simulink model "linearExtendedStateObserver"  (R2021a)
settings: Solver=VariableStepAuto  StartTime=0.0  StopTime=10.0  RelTol=1e-3
settings Model: Creator=krzys  LastModifiedBy=krzys

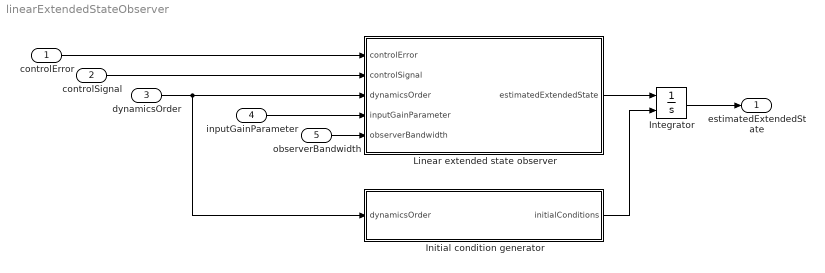
== system linearExtendedStateObserver ==
  controlError : Inport
  controlSignal : Inport  Port=2
  dynamicsOrder : Inport  Port=3
  inputGainParameter : Inport  Port=4
  observerBandwidth : Inport  Port=5
  Initial condition generator : MATLAB Function  TreatAsAtomicUnit=on
  Integrator : Integrator  InitialConditionSource=external
  Linear extended state observer : MATLAB Function  TreatAsAtomicUnit=on
  estimatedExtendedState : Outport
  wires:
  controlError/1 -> Linear extended state observer/1(controlError)
  controlSignal/1 -> Linear extended state observer/2(controlSignal)
  Linear extended state observer/1(estimatedExtendedState) -> Integrator/1
  Integrator/1 -> estimatedExtendedState/1
  dynamicsOrder/1 -> Initial condition generator/1(dynamicsOrder), Linear extended state observer/3(dynamicsOrder)
  inputGainParameter/1 -> Linear extended state observer/4(inputGainParameter)
  observerBandwidth/1 -> Linear extended state observer/5(observerBandwidth)
  Initial condition generator/1(initialConditions) -> Integrator/2

== matlab function linearExtendedStateObserver/Initial condition generator ==
  data: dynamicsOrder input; initialConditions output
function initialConditions = fcn(dynamicsOrder)
    initialConditions = zeros(dynamicsOrder,1);
end

== matlab function linearExtendedStateObserver/Linear extended state observer ==
  data: controlError input; estimatedExtendedState output; controlSignal input; dynamicsOrder input; inputGainParameter input; observerBandwidth input
function estimatedExtendedState = fcn(controlError, controlSignal, dynamicsOrder, inputGainParameter, observerBandwidth)
    
    estimatedExtendedState = 0;
end
